simulink model "gm_lorenz_model_interface"  (R2018a)
settings: Solver=FixedStepAuto  StartTime=0.0  StopTime=inf  RelTol=1e-3  EnableMultiTasking=on
libraries: alterasoclib x12, simulink_extras x1
settings Model: SimulationMode=external  Creator=labuser  LastModifiedBy=labuser
settings SolverCC: ConcurrentTasks=on  PositivePriorityOrder=on  AutoInsertRateTranBlk=on
settings OptimizationCC: BlockReduction=off  ConditionallyExecuteInputs=off  EnhancedBackFolding=on  PassReuseOutputArgsAs=Individual arguments  MaxStackSize=64  OptimizeBlockOrder=speed  DifferentSizesBufferReuse=on  OptimizationCustomize=off
settings DebuggingCC: AlgebraicLoopMsg=error  ParameterTunabilityLossMsg=error
settings HardwareCC: ProdBitPerPointer=32  ProdBitPerSizeT=32  ProdBitPerPtrDiffT=32  ProdLargestAtomicInteger=Long  ProdLargestAtomicFloat=Double  ProdWordSize=32  ProdHWDeviceType=ARM Compatible->ARM Cortex  TargetBitPerPointer=64  TargetBitPerSizeT=64  TargetBitPerPtrDiffT=64  TargetLongLongMode=on  TargetIntDivRoundTo=Zero  TargetEndianess=LittleEndian  TargetWordSize=64  TargetHWDeviceType=Custom Processor->MATLAB Host Computer
settings SFSimCC: MATLABDynamicMemAlloc=off
settings RTWCC: SystemTargetFile=ert.tlc  HardwareBoard=Altera Cyclone V SoC development kit  TLCOptions="-aInlineSetEventsForThisBaseRateFcn=TLC_FALSE -aSuppressMultiTaskScheduler=TLC_FALSE  -aRateBasedStepFcn=0"  TemplateMakefile=ert_default_tmf  GenerateReport=on  Toolchain=ARM Development Studio Altera Edition (DS-5 AE)  IncludeHyperlinkInReport=on  LaunchReport=on  GenerateTraceInfo=on  GenerateTraceReport=on  GenerateTraceReportSl=on  GenerateTraceReportSf=on  GenerateTraceReportEml=on
settings CodeAppCC: ForceParamTrailComments=on  IgnoreCustomStorageClasses=off  OperatorAnnotations=on  SimulinkDataObjDesc=on  SFDataObjDesc=on  InsertBlockDesc=on

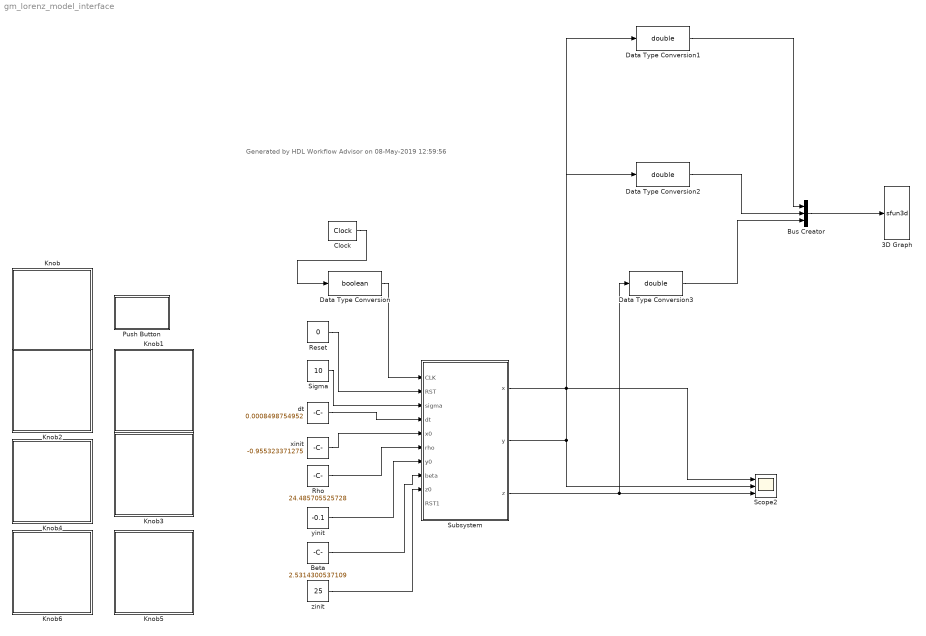
== system gm_lorenz_model_interface ==
  note: Generated by HDL Workflow Advisor on 08-May-2019 12:59:56
  3D Graph : S-Function  LoadFcn=if exist('sfun3d','file'), sfun3d([],[],[],'LoadBlock'); end  FunctionName=sfun3d  Parameters=ax,T,np,cp,gd,ls,mk,mx,hd,tb  SFunctionDeploymentMode=off  EnableBusSupport=off  mask(3D Graph){np=1, ax=[-30 30 -30 30 0 50], mx=2000, T=0.01, cp=[370 -234 -207], gd=on, hd=on, tb=on, ls=-, mk=none}
      mask prompts: np "Number of moving points (lines)"; ax "Range: [xmin xmax  ymin ymax zmin zmax]"; mx "Max number of points in each line"; T "Sampling Time"; cp "Camera position (use [0 0 1] for 2D XY view)"; gd "Grid (on|off)"; hd "HeadMarkers (on|off)"; tb "Toolbar (on|off)"; ls "LineStyle"; mk "LineMarker"
      mask help:
      | This block plots the position of several points in the XYZ space. The input contains the coordinates of all the points (x1,y1,z1,x2,y2,z2,...).
      | The number of moving points (lines), the XYZ ranges, sampling time, camera position, and grid (among other things) can be set as mask parameters.
      settings: CopyFcn=if exist('sfun3d','file'), sfun3d([],[],[],'CopyBlock'); end  DeleteFcn=if exist('sfun3d','file'), sfun3d([],[],[],'DeleteBlock'); end  NameChangeFcn=if exist('sfun3d','file'), sfun3d([],[],[],'NameChange'); end
      mask Help:
      | This block plots the position of several points in the XYZ space. The input contains the coordinates of all the points (x1,y1,z1,x2,y2,z2,...).
      | The number of moving points (lines), the XYZ ranges, sampling time, camera position, and grid (among other things) can be set as mask parameters.
      mask TypeOptions ls: - | -- | : | -. | none
      mask TypeOptions mk: none | . | + | o | * | x | square | diamond | v | ^ | > | < | pentagram | hexagram
      mask Display: plot([.05 .95 .95 .05 .05],[.45 .45 .95 .95 .45], 0.5+cos(0:0.1:2*pi)*0.3,0.7+sin(0:0.1:2*pi)*0.2)
  Beta : Constant  Value=2.5314300537109  OutDataTypeStr=fixdt(1,27,20)  SampleTime=-1
  Bus Creator : BusCreator  Inputs=3
  Clock : simulink_extras/Flip Flops/Clock  period=0.001
  Data Type Conversion : DataTypeConversion  OutDataTypeStr=boolean
  Data Type Conversion1 : DataTypeConversion  OutDataTypeStr=double
  Data Type Conversion2 : DataTypeConversion  OutDataTypeStr=double
  Data Type Conversion3 : DataTypeConversion  OutDataTypeStr=double
  Knob : Subsystem  Description=dt  DialogController=hmiCreateDDGDialog  IsWebBlock=on  mask(MWDashboardBlock){webBlockId=84f497a1-2ba8-42b4-a4e5-becbc4c17d6e, webBlockType=continuousknob, ShowInLibBrowser=on, ShowInitialText=on, HMISrcModelName=gm_lorenz_model_interface}
      mask prompts: webBlockId "WebBlock Id"; webBlockType "WebBlock Type"; HMISrcModelName "Source Model"
      mask help: SimulinkHMI:dialogs:ContinuousKnobDialogDesc
      mask Help: helpview([docroot '/mapfiles/simulink.map'], 'hmi_knob')
      mask Display:
      | if strcmp(get_param(bdroot(gcb),'BlockDiagramType'), 'library')
      |     image([(matlabroot) '/toolbox/simulink/hmi/icons/ContinuousKnob.png']);
      | end
  Knob1 : Subsystem  DialogController=hmiCreateDDGDialog  IsWebBlock=on  mask(MWDashboardBlock){webBlockId=1d3dc13b-7068-47c5-88ea-e950461734b5, webBlockType=continuousknob, ShowInLibBrowser=on, ShowInitialText=on, HMISrcModelName=gm_lorenz_model_interface}
      mask prompts: webBlockId "WebBlock Id"; webBlockType "WebBlock Type"; HMISrcModelName "Source Model"
      mask help: SimulinkHMI:dialogs:ContinuousKnobDialogDesc
      mask Help: helpview([docroot '/mapfiles/simulink.map'], 'hmi_knob')
      mask Display:
      | if strcmp(get_param(bdroot(gcb),'BlockDiagramType'), 'library')
      |     image([(matlabroot) '/toolbox/simulink/hmi/icons/ContinuousKnob.png']);
      | end
  Knob2 : Subsystem  DialogController=hmiCreateDDGDialog  IsWebBlock=on  mask(MWDashboardBlock){webBlockId=03082db3-9890-4786-a189-849826732cd4, webBlockType=continuousknob, ShowInLibBrowser=on, ShowInitialText=on, HMISrcModelName=gm_lorenz_model_interface}
      mask prompts: webBlockId "WebBlock Id"; webBlockType "WebBlock Type"; HMISrcModelName "Source Model"
      mask help: SimulinkHMI:dialogs:ContinuousKnobDialogDesc
      mask Help: helpview([docroot '/mapfiles/simulink.map'], 'hmi_knob')
      mask Display:
      | if strcmp(get_param(bdroot(gcb),'BlockDiagramType'), 'library')
      |     image([(matlabroot) '/toolbox/simulink/hmi/icons/ContinuousKnob.png']);
      | end
  Knob3 : Subsystem  DialogController=hmiCreateDDGDialog  IsWebBlock=on  mask(MWDashboardBlock){webBlockId=28a725e3-ba82-48ed-9f5b-0cbde82ea85c, webBlockType=continuousknob, ShowInLibBrowser=on, ShowInitialText=on, HMISrcModelName=gm_lorenz_model_interface}
      mask prompts: webBlockId "WebBlock Id"; webBlockType "WebBlock Type"; HMISrcModelName "Source Model"
      mask help: SimulinkHMI:dialogs:ContinuousKnobDialogDesc
      mask Help: helpview([docroot '/mapfiles/simulink.map'], 'hmi_knob')
      mask Display:
      | if strcmp(get_param(bdroot(gcb),'BlockDiagramType'), 'library')
      |     image([(matlabroot) '/toolbox/simulink/hmi/icons/ContinuousKnob.png']);
      | end
  Knob4 : Subsystem  DialogController=hmiCreateDDGDialog  IsWebBlock=on  mask(MWDashboardBlock){webBlockId=942013db-1a14-4e6f-80fb-529655d97056, webBlockType=continuousknob, ShowInLibBrowser=on, ShowInitialText=on, HMISrcModelName=gm_lorenz_model_interface}
      mask prompts: webBlockId "WebBlock Id"; webBlockType "WebBlock Type"; HMISrcModelName "Source Model"
      mask help: SimulinkHMI:dialogs:ContinuousKnobDialogDesc
      mask Help: helpview([docroot '/mapfiles/simulink.map'], 'hmi_knob')
      mask Display:
      | if strcmp(get_param(bdroot(gcb),'BlockDiagramType'), 'library')
      |     image([(matlabroot) '/toolbox/simulink/hmi/icons/ContinuousKnob.png']);
      | end
  Knob5 : Subsystem  DialogController=hmiCreateDDGDialog  IsWebBlock=on  mask(MWDashboardBlock){webBlockId=acbfd584-e9fa-4c3e-94ab-875c7d9dd637, webBlockType=continuousknob, ShowInLibBrowser=on, ShowInitialText=on, HMISrcModelName=gm_lorenz_model_interface}
      mask prompts: webBlockId "WebBlock Id"; webBlockType "WebBlock Type"; HMISrcModelName "Source Model"
      mask help: SimulinkHMI:dialogs:ContinuousKnobDialogDesc
      mask Help: helpview([docroot '/mapfiles/simulink.map'], 'hmi_knob')
      mask Display:
      | if strcmp(get_param(bdroot(gcb),'BlockDiagramType'), 'library')
      |     image([(matlabroot) '/toolbox/simulink/hmi/icons/ContinuousKnob.png']);
      | end
  Knob6 : Subsystem  DialogController=hmiCreateDDGDialog  IsWebBlock=on  mask(MWDashboardBlock){webBlockId=48049c15-6c88-4aad-9974-381f7e57f80b, webBlockType=continuousknob, ShowInLibBrowser=on, ShowInitialText=on, HMISrcModelName=gm_lorenz_model_interface}
      mask prompts: webBlockId "WebBlock Id"; webBlockType "WebBlock Type"; HMISrcModelName "Source Model"
      mask help: SimulinkHMI:dialogs:ContinuousKnobDialogDesc
      mask Help: helpview([docroot '/mapfiles/simulink.map'], 'hmi_knob')
      mask Display:
      | if strcmp(get_param(bdroot(gcb),'BlockDiagramType'), 'library')
      |     image([(matlabroot) '/toolbox/simulink/hmi/icons/ContinuousKnob.png']);
      | end
  Push Button : Subsystem  DialogController=hmiCreateDDGDialog  IsWebBlock=on  mask(MWDashboardBlock){webBlockId=15ce415a-1004-47ac-bb23-28b17c9cb58a, webBlockType=pushbutton, ShowInLibBrwoser=on, ShowInitialText=on, HMISrcModelName=gm_lorenz_model_interface}
      mask prompts: webBlockId "WebBlock Id"; webBlockType "WebBlock Type"; HMISrcModelName "Source Model"
      mask help: SimulinkHMI:dialogs:PushButtonDialogDesc
      mask Help: helpview([docroot '/mapfiles/simulink.map'], 'hmi_push_button')
      mask Display:
      | model = bdroot(gcb);
      | if strcmp(get_param(model,'BlockDiagramType'), 'library')
      |     image([(matlabroot) '/toolbox/simulink/hmi/icons/PushButton.png']);
      | end
  Reset : Constant  Value=0  OutDataTypeStr=boolean  SampleTime=-1
  Rho : Constant  Value=24.485705525728  OutDataTypeStr=fixdt(1,27,20)  SampleTime=-1
  Scope2 : Scope  NumInputPorts=3
  Sigma : Constant  Value=10  OutDataTypeStr=fixdt(1,27,20)  SampleTime=-1
  Subsystem : Subsystem  TreatAsAtomicUnit=on  mask(AXI4-Lite/AXI4 Interface){}
      mask help:
      | This is an automatically generated subsystem block.
      | This contains the AXI interface blocks that communicate with the Subsystem_ip IPCore generated from lorenz_model/Subsystem subsystem.
      mask Display: disp(sprintf('Altera SoC \nAXI Interface'));
  dt : Constant  Value=0.0008498754952  OutDataTypeStr=fixdt(1,27,20)  SampleTime=-1
  xinit : Constant  Value=-0.955323371275  OutDataTypeStr=fixdt(1,27,20)  SampleTime=-1
  yinit : Constant  Value=-0.1  OutDataTypeStr=fixdt(1,27,20)  SampleTime=-1
  zinit : Constant  Value=25  OutDataTypeStr=fixdt(1,27,20)  SampleTime=-1
  wires:
  Subsystem/2(y) -> Scope2/2, Data Type Conversion2/1
  Subsystem/3(z) -> Data Type Conversion3/1, Scope2/3
  Subsystem/1(x) -> Scope2/1, Data Type Conversion1/1
  Beta/1 -> Subsystem/8(beta)
  zinit/1 -> Subsystem/9(z0)
  yinit/1 -> Subsystem/7(y0)
  Rho/1 -> Subsystem/6(rho)
  xinit/1 -> Subsystem/5(x0)
  dt/1 -> Subsystem/4(dt)
  Sigma/1 -> Subsystem/3(sigma)
  Data Type Conversion3/1 -> Bus Creator/3
  Data Type Conversion2/1 -> Bus Creator/2
  Data Type Conversion1/1 -> Bus Creator/1
  Bus Creator/1 -> 3D Graph/1
  Data Type Conversion/1 -> Subsystem/1(CLK)
  Clock/1 -> Data Type Conversion/1
  Reset/1 -> Subsystem/2(RST)

== system gm_lorenz_model_interface/Knob ==

== system gm_lorenz_model_interface/Knob1 ==

== system gm_lorenz_model_interface/Knob2 ==

== system gm_lorenz_model_interface/Knob3 ==

== system gm_lorenz_model_interface/Knob4 ==

== system gm_lorenz_model_interface/Knob5 ==

== system gm_lorenz_model_interface/Knob6 ==

== system gm_lorenz_model_interface/Push Button ==

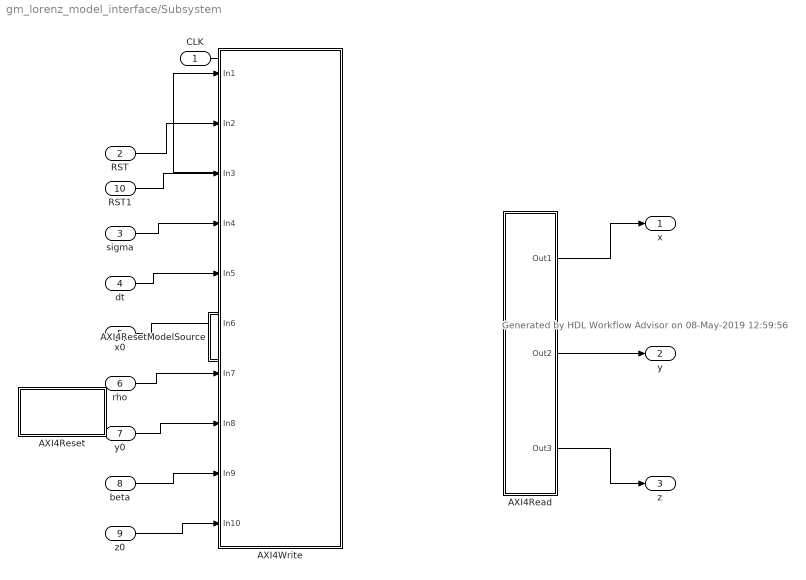
== system gm_lorenz_model_interface/Subsystem ==
  note: Generated by HDL Workflow Advisor on 08-May-2019 12:59:56
  CLK : Inport  OutDataTypeStr=boolean
  RST : Inport  Port=2  OutDataTypeStr=boolean
  sigma : Inport  Port=3  OutDataTypeStr=fixdt(1,27,20)
  dt : Inport  Port=4  OutDataTypeStr=fixdt(1,27,20)
  x0 : Inport  Port=5  OutDataTypeStr=fixdt(1,27,20)
  rho : Inport  Port=6  OutDataTypeStr=fixdt(1,27,20)
  y0 : Inport  Port=7  OutDataTypeStr=fixdt(1,27,20)
  beta : Inport  Port=8  OutDataTypeStr=fixdt(1,27,20)
  z0 : Inport  Port=9  OutDataTypeStr=fixdt(1,27,20)
  RST1 : Inport  Port=10  OutDataTypeStr=boolean
  AXI4Read : Subsystem  Priority=10
  AXI4Reset : Subsystem  mask(System Start){ShowInLibBrowser=0}
      mask prompts: ShowInLibBrowser "Simulink:masks:CustCodeMaskParam1_MP"
      settings: CopyFcn=cccopyfcn(gcb)  OpenFcn=ccopenfcn('System Start Function')
      mask Help: eval('feval(''rtwprivate'',''rtwhelpview'',''rtw_sys_start_block'')');
      mask Display: disp('System\nStart');
  AXI4ResetModelSource : Subsystem  mask(Model Source){ShowInLibBrowser=0}
      mask prompts: ShowInLibBrowser "Simulink:masks:CustCodeMaskParam1_MP"
      settings: CopyFcn=cccopyfcn(gcb)  OpenFcn=ccopenfcn('Model Source')
      mask Help: eval('feval(''rtwprivate'',''rtwhelpview'',''rtw_model_source_block'')');
      mask Display: disp('Model\nSource');
  AXI4Write : Subsystem  Priority=1
  x : Outport  OutDataTypeStr=fixdt(1,27,20)
  y : Outport  Port=2  OutDataTypeStr=fixdt(1,27,20)
  z : Outport  Port=3  OutDataTypeStr=fixdt(1,27,20)
  wires:
  CLK/1 -> AXI4Write/1(In1)
  RST/1 -> AXI4Write/2(In2)
  RST1/1 -> AXI4Write/3(In3)
  sigma/1 -> AXI4Write/4(In4)
  dt/1 -> AXI4Write/5(In5)
  x0/1 -> AXI4Write/6(In6)
  rho/1 -> AXI4Write/7(In7)
  y0/1 -> AXI4Write/8(In8)
  beta/1 -> AXI4Write/9(In9)
  z0/1 -> AXI4Write/10(In10)
  AXI4Read/1(Out1) -> x/1
  AXI4Read/2(Out2) -> y/1
  AXI4Read/3(Out3) -> z/1

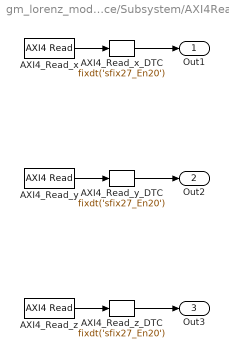
== system gm_lorenz_model_interface/Subsystem/AXI4Read ==
  AXI4_Read_x : alterasoclib/AXI4 Read  Priority=2  DeviceName=/dev/mwipcore  RegisterOffset=hex2dec('124')  DataType=uint32  DataLength=1  SampleTime=-1  BlockPlatform=ALTERASOC
      settings: SourceProductName=Embedded Coder Support Package for Intel SoC Devices  SourceProductBaseCode=EC_ALTERA_SOC
  AXI4_Read_x_DTC : DataTypeConversion  OutDataTypeStr=fixdt('sfix27_En20')  ConvertRealWorld=Stored Integer (SI)
  AXI4_Read_y : alterasoclib/AXI4 Read  Priority=3  DeviceName=/dev/mwipcore  RegisterOffset=hex2dec('128')  DataType=uint32  DataLength=1  SampleTime=-1  BlockPlatform=ALTERASOC
      settings: SourceProductName=Embedded Coder Support Package for Intel SoC Devices  SourceProductBaseCode=EC_ALTERA_SOC
  AXI4_Read_y_DTC : DataTypeConversion  OutDataTypeStr=fixdt('sfix27_En20')  ConvertRealWorld=Stored Integer (SI)
  AXI4_Read_z : alterasoclib/AXI4 Read  Priority=4  DeviceName=/dev/mwipcore  RegisterOffset=hex2dec('12C')  DataType=uint32  DataLength=1  SampleTime=-1  BlockPlatform=ALTERASOC
      settings: SourceProductName=Embedded Coder Support Package for Intel SoC Devices  SourceProductBaseCode=EC_ALTERA_SOC
  AXI4_Read_z_DTC : DataTypeConversion  OutDataTypeStr=fixdt('sfix27_En20')  ConvertRealWorld=Stored Integer (SI)
  Out1 : Outport
  Out2 : Outport  Port=2
  Out3 : Outport  Port=3
  wires:
  AXI4_Read_y_DTC/1 -> Out2/1
  AXI4_Read_y/1 -> AXI4_Read_y_DTC/1
  AXI4_Read_x/1 -> AXI4_Read_x_DTC/1
  AXI4_Read_x_DTC/1 -> Out1/1
  AXI4_Read_z/1 -> AXI4_Read_z_DTC/1
  AXI4_Read_z_DTC/1 -> Out3/1

== system gm_lorenz_model_interface/Subsystem/AXI4Reset ==

== system gm_lorenz_model_interface/Subsystem/AXI4ResetModelSource ==

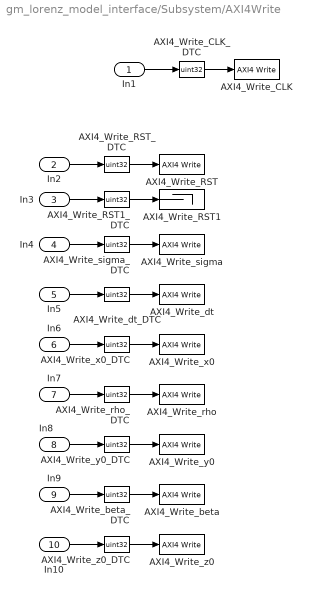
== system gm_lorenz_model_interface/Subsystem/AXI4Write ==
  In1 : Inport
  In2 : Inport  Port=2
  In3 : Inport  Port=3
  In4 : Inport  Port=4
  In5 : Inport  Port=5
  In6 : Inport  Port=6
  In7 : Inport  Port=7
  In8 : Inport  Port=8
  In9 : Inport  Port=9
  In10 : Inport  Port=10
  AXI4_Write_CLK : alterasoclib/AXI4 Write  Priority=1  DeviceName=/dev/mwipcore  RegisterOffset=hex2dec('100')  BlockPlatform=ALTERASOC
      settings: SourceProductName=Embedded Coder Support Package for Intel SoC Devices  SourceProductBaseCode=EC_ALTERA_SOC
  AXI4_Write_CLK_DTC : DataTypeConversion  OutDataTypeStr=uint32  ConvertRealWorld=Stored Integer (SI)
  AXI4_Write_RST : alterasoclib/AXI4 Write  Priority=2  DeviceName=/dev/mwipcore  RegisterOffset=hex2dec('104')  BlockPlatform=ALTERASOC
      settings: SourceProductName=Embedded Coder Support Package for Intel SoC Devices  SourceProductBaseCode=EC_ALTERA_SOC
  AXI4_Write_RST1 : Terminator
  AXI4_Write_RST1_DTC : DataTypeConversion  OutDataTypeStr=uint32  ConvertRealWorld=Stored Integer (SI)
  AXI4_Write_RST_DTC : DataTypeConversion  OutDataTypeStr=uint32  ConvertRealWorld=Stored Integer (SI)
  AXI4_Write_beta : alterasoclib/AXI4 Write  Priority=8  DeviceName=/dev/mwipcore  RegisterOffset=hex2dec('11C')  BlockPlatform=ALTERASOC
      settings: SourceProductName=Embedded Coder Support Package for Intel SoC Devices  SourceProductBaseCode=EC_ALTERA_SOC
  AXI4_Write_beta_DTC : DataTypeConversion  OutDataTypeStr=uint32  ConvertRealWorld=Stored Integer (SI)
  AXI4_Write_dt : alterasoclib/AXI4 Write  Priority=4  DeviceName=/dev/mwipcore  RegisterOffset=hex2dec('10C')  BlockPlatform=ALTERASOC
      settings: SourceProductName=Embedded Coder Support Package for Intel SoC Devices  SourceProductBaseCode=EC_ALTERA_SOC
  AXI4_Write_dt_DTC : DataTypeConversion  OutDataTypeStr=uint32  ConvertRealWorld=Stored Integer (SI)
  AXI4_Write_rho : alterasoclib/AXI4 Write  Priority=6  DeviceName=/dev/mwipcore  RegisterOffset=hex2dec('114')  BlockPlatform=ALTERASOC
      settings: SourceProductName=Embedded Coder Support Package for Intel SoC Devices  SourceProductBaseCode=EC_ALTERA_SOC
  AXI4_Write_rho_DTC : DataTypeConversion  OutDataTypeStr=uint32  ConvertRealWorld=Stored Integer (SI)
  AXI4_Write_sigma : alterasoclib/AXI4 Write  Priority=3  DeviceName=/dev/mwipcore  RegisterOffset=hex2dec('108')  BlockPlatform=ALTERASOC
      settings: SourceProductName=Embedded Coder Support Package for Intel SoC Devices  SourceProductBaseCode=EC_ALTERA_SOC
  AXI4_Write_sigma_DTC : DataTypeConversion  OutDataTypeStr=uint32  ConvertRealWorld=Stored Integer (SI)
  AXI4_Write_x0 : alterasoclib/AXI4 Write  Priority=5  DeviceName=/dev/mwipcore  RegisterOffset=hex2dec('110')  BlockPlatform=ALTERASOC
      settings: SourceProductName=Embedded Coder Support Package for Intel SoC Devices  SourceProductBaseCode=EC_ALTERA_SOC
  AXI4_Write_x0_DTC : DataTypeConversion  OutDataTypeStr=uint32  ConvertRealWorld=Stored Integer (SI)
  AXI4_Write_y0 : alterasoclib/AXI4 Write  Priority=7  DeviceName=/dev/mwipcore  RegisterOffset=hex2dec('118')  BlockPlatform=ALTERASOC
      settings: SourceProductName=Embedded Coder Support Package for Intel SoC Devices  SourceProductBaseCode=EC_ALTERA_SOC
  AXI4_Write_y0_DTC : DataTypeConversion  OutDataTypeStr=uint32  ConvertRealWorld=Stored Integer (SI)
  AXI4_Write_z0 : alterasoclib/AXI4 Write  Priority=9  DeviceName=/dev/mwipcore  RegisterOffset=hex2dec('120')  BlockPlatform=ALTERASOC
      settings: SourceProductName=Embedded Coder Support Package for Intel SoC Devices  SourceProductBaseCode=EC_ALTERA_SOC
  AXI4_Write_z0_DTC : DataTypeConversion  OutDataTypeStr=uint32  ConvertRealWorld=Stored Integer (SI)
  wires:
  AXI4_Write_z0_DTC/1 -> AXI4_Write_z0/1
  AXI4_Write_y0_DTC/1 -> AXI4_Write_y0/1
  AXI4_Write_dt_DTC/1 -> AXI4_Write_dt/1
  AXI4_Write_sigma_DTC/1 -> AXI4_Write_sigma/1
  AXI4_Write_x0_DTC/1 -> AXI4_Write_x0/1
  AXI4_Write_beta_DTC/1 -> AXI4_Write_beta/1
  AXI4_Write_rho_DTC/1 -> AXI4_Write_rho/1
  In9/1 -> AXI4_Write_beta_DTC/1
  AXI4_Write_CLK_DTC/1 -> AXI4_Write_CLK/1
  In2/1 -> AXI4_Write_RST_DTC/1
  AXI4_Write_RST_DTC/1 -> AXI4_Write_RST/1
  AXI4_Write_RST1_DTC/1 -> AXI4_Write_RST1/1
  In1/1 -> AXI4_Write_CLK_DTC/1
  In5/1 -> AXI4_Write_dt_DTC/1
  In3/1 -> AXI4_Write_RST1_DTC/1
  In6/1 -> AXI4_Write_x0_DTC/1
  In4/1 -> AXI4_Write_sigma_DTC/1
  In7/1 -> AXI4_Write_rho_DTC/1
  In8/1 -> AXI4_Write_y0_DTC/1
  In10/1 -> AXI4_Write_z0_DTC/1
